simulink model "mrefrobotarm_modified_previous_y_previous_u_previous_ref_prepro"  (R2018b)
settings: Solver=FixedStepAuto  StartTime=0.0  StopTime=10  RelTol=1e-3  AbsTol=1e-6
undefined symbols (not defined in the file or in its folder): cc, options
libraries: neural x594, simulink x1
(part 6 of 22)

== system mrefrobotarm_modified_previous_y_previous_u_previous_ref_prepro/m=0.01 sd =0.01/Layer 3/Delays 1 ==
  "p{3}" : Inport  PortDimensions=30
      mask Display: e = 0.06;c1 = [120 230 180]/255;c2 = ([120 230 180]+0)/(256+128);c3 = ([120 230 180]+128)/(256+128);patch([0 1 1 0],[0 0 1 1],c1);patch([0 1 1 1-e 1-e 0+e],[0 0 1 1-e 0+e 0+e],c2);patch([0 0 1 1-e 0+e 0+e],[0 1 1 1-e 1-e 0+e],c3);plot([0 1 1 0 0],[0 0 1 1 0]);
  mux : Mux  Inputs=1
      mask Display: e = 0.06;c1 = [120 150 230]/255;c2 = ([120 150 230]+0)/383;c3 = ([120 150 230]+128)/383;patch([0 1 1 0],[0 0 1 1],c1);patch([0 1 1 1-e 1-e 0+e],[0 0 1 1-e 0+e 0+e],c2);patch([0 0 1 1-e 0+e 0+e],[0 1 1 1-e 1-e 0+e],c3);plot([0 1 1 0 0],[0 0 1 1 0]);disp('Mux')
  "pd{3,2}" : Outport
      mask Display: e = 0.06;c1 = [120 230 180]/255;c2 = ([120 230 180]+0)/(256+128);c3 = ([120 230 180]+128)/(256+128);patch([0 1 1 0],[0 0 1 1],c1);patch([0 1 1 1-e 1-e 0+e],[0 0 1 1-e 0+e 0+e],c2);patch([0 0 1 1-e 0+e 0+e],[0 1 1 1-e 1-e 0+e],c3);plot([0 1 1 0 0],[0 0 1 1 0]);
  wires:
  "p{3}"/1 -> mux/1
  mux/1 -> "pd{3,2}"/1

== system mrefrobotarm_modified_previous_y_previous_u_previous_ref_prepro/m=0.01 sd =0.01/Layer 3/LW{3,2} ==
  "ad{3,2}" : Inport  PortDimensions=30
      mask Display: e = 0.06;c1 = [120 230 180]/255;c2 = ([120 230 180]+0)/(256+128);c3 = ([120 230 180]+128)/(256+128);patch([0 1 1 0],[0 0 1 1],c1);patch([0 1 1 1-e 1-e 0+e],[0 0 1 1-e 0+e 0+e],c2);patch([0 0 1 1-e 0+e 0+e],[0 1 1 1-e 1-e 0+e],c3);plot([0 1 1 0 0],[0 0 1 1 0]);
  "IW{3,2}(1,:)'" : Constant  Value=[0.0028381381201219024745796559727750718593597412109375;-0.00708260609535531389380214051243456196971237659454345703125;-0.00583488335220346855669593111315407440997660160064697265625;0.01020530930108067869943599959015045897103846073150634765625;0.0035026247420214058798937362126935113337822258472442626953125;0.007372665491954556553355626391521582263521850109100341796875;0.0082512842468972780185509918737807311117649078369140625;-0.006754245741655124334046345069282324402593076229095458984375;0.001683452101721956591096063249324288335628807544708251953125;-0.00690829099421421365112561119303791201673448085784912109375;0.01314880348478297822367721892078407108783721923828125;-0.007470263091506845927469715462621024926193058490753173828125;-0.00542419932097103381363201179965471965260803699493408203125;-0.01146260049752216743368382623202705872245132923126220703125;-0.009116602607925426704493787610772415064275264739990234375;-0.0032803912590090062058323372440327148069627583026885986328125;-0.006661633151908582205213971150215002126060426235198974609375;-0.0289839272926558366716420778175233863294124603271484375;0.007080157965975715332607176577539576101116836071014404296875;1.106395796742202453089021219057030975818634033203125;0.0098157682894019597508172836342055234126746654510498046875;-0.00914110666628639191577665457089096889831125736236572265625;-0.00060787204210546621867272687467220748658291995525360107421875;-0.00883143986489790498717322719812727882526814937591552734375;0.0082676478536601351321255748416660935617983341217041015625;-0.00932936505581516591079083156046181102283298969268798828125;-0.00127195106162408637373584241458956967107951641082763671875;-0.00692592170297301294723535391995028476230800151824951171875;0.009542106880190574791367197349245543591678142547607421875;-0.00879287702148130560775296515885202097706496715545654296875]
      mask Display: e = 0.06;c1 = [120 150 230]/255;c2 = ([120 150 230]+0)/383;c3 = ([120 150 230]+128)/383;patch([0 1 1 0],[0 0 1 1],c1);patch([0 1 1 1-e 1-e 0+e],[0 0 1 1-e 0+e 0+e],c2);patch([0 0 1 1-e 0+e 0+e],[0 1 1 1-e 1-e 0+e],c3);plot([0 1 1 0 0],[0 0 1 1 0]);disp('weights');
  Mux : Mux  Inputs=1
      mask Display: e = 0.06;c1 = [120 150 230]/255;c2 = ([120 150 230]+0)/383;c3 = ([120 150 230]+128)/383;patch([0 1 1 0],[0 0 1 1],c1);patch([0 1 1 1-e 1-e 0+e],[0 0 1 1-e 0+e 0+e],c2);patch([0 0 1 1-e 0+e 0+e],[0 1 1 1-e 1-e 0+e],c3);plot([0 1 1 0 0],[0 0 1 1 0]);disp('Mux');
  dotprod1 : neural/Weight Functions/dotprod
  "lz{3,2}" : Outport
      mask Display: e = 0.06;c1 = [120 230 180]/255;c2 = ([120 230 180]+0)/(256+128);c3 = ([120 230 180]+128)/(256+128);patch([0 1 1 0],[0 0 1 1],c1);patch([0 1 1 1-e 1-e 0+e],[0 0 1 1-e 0+e 0+e],c2);patch([0 0 1 1-e 0+e 0+e],[0 1 1 1-e 1-e 0+e],c3);plot([0 1 1 0 0],[0 0 1 1 0]);
  wires:
  "IW{3,2}(1,:)'"/1 -> dotprod1/1
  "ad{3,2}"/1 -> dotprod1/2
  dotprod1/1 -> Mux/1
  Mux/1 -> "lz{3,2}"/1

== system mrefrobotarm_modified_previous_y_previous_u_previous_ref_prepro/pre_0/Layer 1/Delays 1 ==
  "p{1}" : Inport  PortDimensions=10
      mask Display: e = 0.06;c1 = [120 230 180]/255;c2 = ([120 230 180]+0)/(256+128);c3 = ([120 230 180]+128)/(256+128);patch([0 1 1 0],[0 0 1 1],c1);patch([0 1 1 1-e 1-e 0+e],[0 0 1 1-e 0+e 0+e],c2);patch([0 0 1 1-e 0+e 0+e],[0 1 1 1-e 1-e 0+e],c3);plot([0 1 1 0 0],[0 0 1 1 0]);
  mux : Mux  Inputs=1
      mask Display: e = 0.06;c1 = [120 150 230]/255;c2 = ([120 150 230]+0)/383;c3 = ([120 150 230]+128)/383;patch([0 1 1 0],[0 0 1 1],c1);patch([0 1 1 1-e 1-e 0+e],[0 0 1 1-e 0+e 0+e],c2);patch([0 0 1 1-e 0+e 0+e],[0 1 1 1-e 1-e 0+e],c3);plot([0 1 1 0 0],[0 0 1 1 0]);disp('Mux')
  "pd{1,1}" : Outport
      mask Display: e = 0.06;c1 = [120 230 180]/255;c2 = ([120 230 180]+0)/(256+128);c3 = ([120 230 180]+128)/(256+128);patch([0 1 1 0],[0 0 1 1],c1);patch([0 1 1 1-e 1-e 0+e],[0 0 1 1-e 0+e 0+e],c2);patch([0 0 1 1-e 0+e 0+e],[0 1 1 1-e 1-e 0+e],c3);plot([0 1 1 0 0],[0 0 1 1 0]);
  wires:
  "p{1}"/1 -> mux/1
  mux/1 -> "pd{1,1}"/1

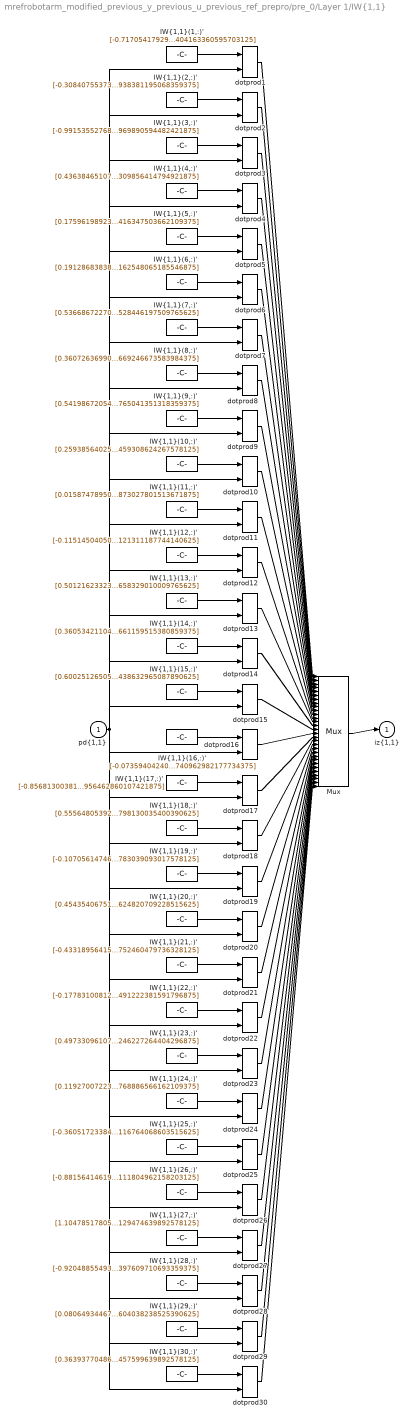
== system mrefrobotarm_modified_previous_y_previous_u_previous_ref_prepro/pre_0/Layer 1/IW{1,1} ==
  "pd{1,1}" : Inport  PortDimensions=10
      mask Display: e = 0.06;c1 = [120 230 180]/255;c2 = ([120 230 180]+0)/(256+128);c3 = ([120 230 180]+128)/(256+128);patch([0 1 1 0],[0 0 1 1],c1);patch([0 1 1 1-e 1-e 0+e],[0 0 1 1-e 0+e 0+e],c2);patch([0 0 1 1-e 0+e 0+e],[0 1 1 1-e 1-e 0+e],c3);plot([0 1 1 0 0],[0 0 1 1 0]);
  "IW{1,1}(1,:)'" : Constant  Value=[-0.7170541792926499180538257860462181270122528076171875;-0.53730470878595426587054362244089134037494659423828125;0.85386649215660692657792196769150905311107635498046875;-0.439278400220474873894005440888577140867710113525390625;0.338061858528379610699943214058293960988521575927734375;0.28368532083581954328366236950387246906757354736328125;-0.961821049186493581828472088091075420379638671875;-0.49782743481612723446261270510149188339710235595703125;-0.0877755253396242662855541993849328719079494476318359375;0.180319748256219380966314247416448779404163360595703125]
      mask Display: e = 0.06;c1 = [120 150 230]/255;c2 = ([120 150 230]+0)/383;c3 = ([120 150 230]+128)/383;patch([0 1 1 0],[0 0 1 1],c1);patch([0 1 1 1-e 1-e 0+e],[0 0 1 1-e 0+e 0+e],c2);patch([0 0 1 1-e 0+e 0+e],[0 1 1 1-e 1-e 0+e],c3);plot([0 1 1 0 0],[0 0 1 1 0]);disp('Weights');
  "IW{1,1}(10,:)'" : Constant  Value=[0.25938564025182764272159374741022475063800811767578125;-0.5066291721836615469243270126753486692905426025390625;0.365194749586469746827077642592485062777996063232421875;0.34016798405581039066447601726395078003406524658203125;0.73685097441923164129917722675600089132785797119140625;0.77610806782460539654522335695219226181507110595703125;-0.89757418772604735668352304855943657457828521728515625;0.30341865744586205000388190455851145088672637939453125;0.4921579361872365776520155122852884232997894287109375;-0.635709476416032703838254747097380459308624267578125]
      mask Display: e = 0.06;c1 = [120 150 230]/255;c2 = ([120 150 230]+0)/383;c3 = ([120 150 230]+128)/383;patch([0 1 1 0],[0 0 1 1],c1);patch([0 1 1 1-e 1-e 0+e],[0 0 1 1-e 0+e 0+e],c2);patch([0 0 1 1-e 0+e 0+e],[0 1 1 1-e 1-e 0+e],c3);plot([0 1 1 0 0],[0 0 1 1 0]);disp('Weights');
  "IW{1,1}(11,:)'" : Constant  Value=[0.015874789502760534853909035746255540288984775543212890625;0.462275145120222108463536869749077595770359039306640625;0.0032692520327777508347411039579810676514171063899993896484375;0.05251953017595435702080663986635045148432254791259765625;0.91141322247884082319302478936151601374149322509765625;-0.79281915938791136522212354975636117160320281982421875;-0.4515989926503818363556774784228764474391937255859375;0.9314165577462818479403949822881259024143218994140625;-0.261347523270411274953772817752906121313571929931640625;-0.10546819823597312903995515398491988889873027801513671875]
      mask Display: e = 0.06;c1 = [120 150 230]/255;c2 = ([120 150 230]+0)/383;c3 = ([120 150 230]+128)/383;patch([0 1 1 0],[0 0 1 1],c1);patch([0 1 1 1-e 1-e 0+e],[0 0 1 1-e 0+e 0+e],c2);patch([0 0 1 1-e 0+e 0+e],[0 1 1 1-e 1-e 0+e],c3);plot([0 1 1 0 0],[0 0 1 1 0]);disp('Weights');
  "IW{1,1}(12,:)'" : Constant  Value=[-0.11514504050898012599279951473363325931131839752197265625;0.813469898806353786113731985096819698810577392578125;0.490011957774175499480406870134174823760986328125;0.164969195990666117612732932684593833982944488525390625;-0.85432220477327092122976637256215326488018035888671875;-0.57011847095452872213883210861240513622760772705078125;0.288064489380212174207684938664897345006465911865234375;0.2419661153783553009244400300303823314607143402099609375;0.311681589957975513360821651076548732817173004150390625;-0.1664504145084248210029187475811340846121311187744140625]
      mask Display: e = 0.06;c1 = [120 150 230]/255;c2 = ([120 150 230]+0)/383;c3 = ([120 150 230]+128)/383;patch([0 1 1 0],[0 0 1 1],c1);patch([0 1 1 1-e 1-e 0+e],[0 0 1 1-e 0+e 0+e],c2);patch([0 0 1 1-e 0+e 0+e],[0 1 1 1-e 1-e 0+e],c3);plot([0 1 1 0 0],[0 0 1 1 0]);disp('Weights');
  "IW{1,1}(13,:)'" : Constant  Value=[0.50121623323530239968448540821555070579051971435546875;-0.7679058675490575414102067952626384794712066650390625;0.2332901346448288670831772151359473355114459991455078125;-0.05845892447780610956531432975680218078196048736572265625;-0.52276177164686721265951518944348208606243133544921875;1.161972018816590068723826334462501108646392822265625;0.10355864424138964963173492606074432842433452606201171875;-0.64286579959598366684758730116300284862518310546875;0.3284995499970400079092769374256022274494171142578125;0.667607800202736800798675176338292658329010009765625]
      mask Display: e = 0.06;c1 = [120 150 230]/255;c2 = ([120 150 230]+0)/383;c3 = ([120 150 230]+128)/383;patch([0 1 1 0],[0 0 1 1],c1);patch([0 1 1 1-e 1-e 0+e],[0 0 1 1-e 0+e 0+e],c2);patch([0 0 1 1-e 0+e 0+e],[0 1 1 1-e 1-e 0+e],c3);plot([0 1 1 0 0],[0 0 1 1 0]);disp('Weights');
  "IW{1,1}(14,:)'" : Constant  Value=[0.36053421104863614399249627240351401269435882568359375;-0.1762721064183007946279957423030282370746135711669921875;0.251082557900824177021803507159347645938396453857421875;0.020135728323763042724170446717835147865116596221923828125;-0.85072127871646829877505524564185179769992828369140625;0.84743056157007234929778860532678663730621337890625;-0.945997916723647858106005514855496585369110107421875;0.94095072199429896642186577082611620426177978515625;-0.249932980099258295059172496621613390743732452392578125;0.2125377599592276067763663149889907799661159515380859375]
      mask Display: e = 0.06;c1 = [120 150 230]/255;c2 = ([120 150 230]+0)/383;c3 = ([120 150 230]+128)/383;patch([0 1 1 0],[0 0 1 1],c1);patch([0 1 1 1-e 1-e 0+e],[0 0 1 1-e 0+e 0+e],c2);patch([0 0 1 1-e 0+e 0+e],[0 1 1 1-e 1-e 0+e],c3);plot([0 1 1 0 0],[0 0 1 1 0]);disp('Weights');
  "IW{1,1}(15,:)'" : Constant  Value=[0.60025126505590609138351965157198719680309295654296875;-0.66688231279006193741309971301234327256679534912109375;-0.91654840056374220491619553286000154912471771240234375;-0.471001673909513030036322334126452915370464324951171875;0.53790409729519372827866163788712583482265472412109375;0.5322213146726231247640725996461696922779083251953125;0.138282833645754166251862216086010448634624481201171875;-0.77416314549115250454036640803678892552852630615234375;-0.5552894515247055462481284848763607442378997802734375;0.1648030102917383832306086333119310438632965087890625]
      mask Display: e = 0.06;c1 = [120 150 230]/255;c2 = ([120 150 230]+0)/383;c3 = ([120 150 230]+128)/383;patch([0 1 1 0],[0 0 1 1],c1);patch([0 1 1 1-e 1-e 0+e],[0 0 1 1-e 0+e 0+e],c2);patch([0 0 1 1-e 0+e 0+e],[0 1 1 1-e 1-e 0+e],c3);plot([0 1 1 0 0],[0 0 1 1 0]);disp('Weights');
  "IW{1,1}(16,:)'" : Constant  Value=[-0.0735940424037289375736037300157477147877216339111328125;0.12992241719517527709371051969355903565883636474609375;0.3713405142616206244809973213705234229564666748046875;0.1763399041436344572009176090432447381317615509033203125;-0.05111110475284337539836343466959078796207904815673828125;0.460151189735468924002503854353562928736209869384765625;0.7322632127881096852917153228190727531909942626953125;-1.007932226242228779256038251332938671112060546875;0.77228494687098148130388608478824608027935028076171875;-0.37142538987047879484038048758520744740962982177734375]
      mask Display: e = 0.06;c1 = [120 150 230]/255;c2 = ([120 150 230]+0)/383;c3 = ([120 150 230]+128)/383;patch([0 1 1 0],[0 0 1 1],c1);patch([0 1 1 1-e 1-e 0+e],[0 0 1 1-e 0+e 0+e],c2);patch([0 0 1 1-e 0+e 0+e],[0 1 1 1-e 1-e 0+e],c3);plot([0 1 1 0 0],[0 0 1 1 0]);disp('Weights');
  "IW{1,1}(17,:)'" : Constant  Value=[-0.85681300381991631898159766933531500399112701416015625;-0.53097179335189592652710643960745073854923248291015625;1.01247292983426628865117891109548509120941162109375;0.378991230739149143058597246636054478585720062255859375;0.294378095574322984351312015860457904636859893798828125;-0.602953992325712562205808353610336780548095703125;-0.56336544113835262947986848303116858005523681640625;0.90595353858253113710219395215972326695919036865234375;0.57769092650718534276421678441693075001239776611328125;0.89314033041056084538666937078232876956462860107421875]
      mask Display: e = 0.06;c1 = [120 150 230]/255;c2 = ([120 150 230]+0)/383;c3 = ([120 150 230]+128)/383;patch([0 1 1 0],[0 0 1 1],c1);patch([0 1 1 1-e 1-e 0+e],[0 0 1 1-e 0+e 0+e],c2);patch([0 0 1 1-e 0+e 0+e],[0 1 1 1-e 1-e 0+e],c3);plot([0 1 1 0 0],[0 0 1 1 0]);disp('Weights');
  "IW{1,1}(18,:)'" : Constant  Value=[0.555648053924087559352074094931595027446746826171875;0.504375695640225440996573524898849427700042724609375;-0.333632718241962333838301901778322644531726837158203125;0.5008843209308257993228608029312454164028167724609375;-0.237702821178001288959791281740763224661350250244140625;-0.7162760582970670864000339861377142369747161865234375;0.51637313021700015358561586253927089273929595947265625;0.173311238874638118279136733690393157303333282470703125;-0.7997650713717643355948894168250262737274169921875;-0.8738812033958078817619252731674350798130035400390625]
      mask Display: e = 0.06;c1 = [120 150 230]/255;c2 = ([120 150 230]+0)/383;c3 = ([120 150 230]+128)/383;patch([0 1 1 0],[0 0 1 1],c1);patch([0 1 1 1-e 1-e 0+e],[0 0 1 1-e 0+e 0+e],c2);patch([0 0 1 1-e 0+e 0+e],[0 1 1 1-e 1-e 0+e],c3);plot([0 1 1 0 0],[0 0 1 1 0]);disp('Weights');
  "IW{1,1}(19,:)'" : Constant  Value=[-0.10705614746581405827274835473872371949255466461181640625;0.1487441877660455047394094663104624487459659576416015625;-0.26390898079033842105189933135989122092723846435546875;-0.6493337689871576667854924380662851035594940185546875;-0.46145541066660289430956254363991320133209228515625;-0.142170787004473997416909014646080322563648223876953125;1.012033043287881017846530085080303251743316650390625;-0.319071927015635414814909154301858507096767425537109375;-0.516709582947004530950607659178785979747772216796875;0.50320529256654034089280003172461874783039093017578125]
      mask Display: e = 0.06;c1 = [120 150 230]/255;c2 = ([120 150 230]+0)/383;c3 = ([120 150 230]+128)/383;patch([0 1 1 0],[0 0 1 1],c1);patch([0 1 1 1-e 1-e 0+e],[0 0 1 1-e 0+e 0+e],c2);patch([0 0 1 1-e 0+e 0+e],[0 1 1 1-e 1-e 0+e],c3);plot([0 1 1 0 0],[0 0 1 1 0]);disp('Weights');
  "IW{1,1}(2,:)'" : Constant  Value=[-0.30840755373511308246037287972285412251949310302734375;-0.099084112890050535238373186075477860867977142333984375;0.81717661091166771125671175468596629798412322998046875;-0.6092062881178741395871156782959587872028350830078125;-0.50860553050792145501901586612802930176258087158203125;-0.6625835472015584315386149683035910129547119140625;0.75851058462894760392458692876971326768398284912109375;-0.037532246529271333368438234856512281112372875213623046875;0.79511476519777823934731486588134430348873138427734375;0.37191656633381453556097540058544836938381195068359375]
      mask Display: e = 0.06;c1 = [120 150 230]/255;c2 = ([120 150 230]+0)/383;c3 = ([120 150 230]+128)/383;patch([0 1 1 0],[0 0 1 1],c1);patch([0 1 1 1-e 1-e 0+e],[0 0 1 1-e 0+e 0+e],c2);patch([0 0 1 1-e 0+e 0+e],[0 1 1 1-e 1-e 0+e],c3);plot([0 1 1 0 0],[0 0 1 1 0]);disp('Weights');
  "IW{1,1}(20,:)'" : Constant  Value=[0.454354067516998527676008734488277696073055267333984375;0.57137295812917321402579773348406888544559478759765625;-0.1850233688088059047505140597422723658382892608642578125;0.386724997843112927586872729079914279282093048095703125;0.039258849478771173924229742624447681009769439697265625;0.67472078143233493729979954878217540681362152099609375;0.92573329751093591521993175774696283042430877685546875;-0.70208984056181711341793061365024186670780181884765625;-0.7554651342448270856522185567882843315601348876953125;-0.653164724819280451129088760353624820709228515625]
      mask Display: e = 0.06;c1 = [120 150 230]/255;c2 = ([120 150 230]+0)/383;c3 = ([120 150 230]+128)/383;patch([0 1 1 0],[0 0 1 1],c1);patch([0 1 1 1-e 1-e 0+e],[0 0 1 1-e 0+e 0+e],c2);patch([0 0 1 1-e 0+e 0+e],[0 1 1 1-e 1-e 0+e],c3);plot([0 1 1 0 0],[0 0 1 1 0]);disp('Weights');
  "IW{1,1}(21,:)'" : Constant  Value=[-0.4331895641543983543897411436773836612701416015625;0.8989764475014252465001618475071154534816741943359375;-0.54666182104691929399820082835503853857517242431640625;-0.56008518072537050169756867035175673663616180419921875;-0.177121978724637030300215201350511051714420318603515625;-0.9354064903881589287948372657410800457000732421875;0.5262284428804051561456844865460880100727081298828125;0.638291312447713199418330987100489437580108642578125;-0.372536639664820812267720384625135920941829681396484375;-0.60323093663160876065632010067929513752460479736328125]
      mask Display: e = 0.06;c1 = [120 150 230]/255;c2 = ([120 150 230]+0)/383;c3 = ([120 150 230]+128)/383;patch([0 1 1 0],[0 0 1 1],c1);patch([0 1 1 1-e 1-e 0+e],[0 0 1 1-e 0+e 0+e],c2);patch([0 0 1 1-e 0+e 0+e],[0 1 1 1-e 1-e 0+e],c3);plot([0 1 1 0 0],[0 0 1 1 0]);disp('Weights');
  "IW{1,1}(22,:)'" : Constant  Value=[-0.1778310081286245125653522336506284773349761962890625;-0.58116958910897731360734042027615942060947418212890625;0.76548783415328924828457957119098864495754241943359375;0.311107618873479319088204420040710829198360443115234375;-0.03968922139101148383044659340157522819936275482177734375;-0.843995838711065093917795820743776857852935791015625;0.206526298912914629823944778763689100742340087890625;-0.359170465722282561404909984048572368919849395751953125;0.5525388023226003308963072413462214171886444091796875;1.0572457569624578166411765778320841491222381591796875]
      mask Display: e = 0.06;c1 = [120 150 230]/255;c2 = ([120 150 230]+0)/383;c3 = ([120 150 230]+128)/383;patch([0 1 1 0],[0 0 1 1],c1);patch([0 1 1 1-e 1-e 0+e],[0 0 1 1-e 0+e 0+e],c2);patch([0 0 1 1-e 0+e 0+e],[0 1 1 1-e 1-e 0+e],c3);plot([0 1 1 0 0],[0 0 1 1 0]);disp('Weights');
  "IW{1,1}(23,:)'" : Constant  Value=[0.49733096107312502187625113947433419525623321533203125;0.89927052734582202386803828630945645272731781005859375;-0.0394225177103877388873343079467304050922393798828125;-0.57836371627708604847839524154551327228546142578125;0.1021461496097287591222624314468703232705593109130859375;0.038811398906852888346374896855195402167737483978271484375;0.2188587004529818080822423098652507178485393524169921875;0.28864377705730703826958460922469384968280792236328125;-0.11510758072953168607011065205369959585368633270263671875;-1.082554482942160500869022143888287246227264404296875]
      mask Display: e = 0.06;c1 = [120 150 230]/255;c2 = ([120 150 230]+0)/383;c3 = ([120 150 230]+128)/383;patch([0 1 1 0],[0 0 1 1],c1);patch([0 1 1 1-e 1-e 0+e],[0 0 1 1-e 0+e 0+e],c2);patch([0 0 1 1-e 0+e 0+e],[0 1 1 1-e 1-e 0+e],c3);plot([0 1 1 0 0],[0 0 1 1 0]);disp('Weights');
  "IW{1,1}(24,:)'" : Constant  Value=[0.11927007223421805248708693625303567387163639068603515625;-0.78217240703766410803154940367676317691802978515625;0.79957722702048228402560425820411182940006256103515625;-0.68075308000872591929208965666475705802440643310546875;0.67785256439370822345580336332204751670360565185546875;-0.46377662029388100339843958863639272749423980712890625;-0.7071229604349558162112998616066761314868927001953125;0.32062142479983446463620566646568477153778076171875;1.0306127438644454574756537112989462912082672119140625;0.474999448772362276027791949672973714768886566162109375]
      mask Display: e = 0.06;c1 = [120 150 230]/255;c2 = ([120 150 230]+0)/383;c3 = ([120 150 230]+128)/383;patch([0 1 1 0],[0 0 1 1],c1);patch([0 1 1 1-e 1-e 0+e],[0 0 1 1-e 0+e 0+e],c2);patch([0 0 1 1-e 0+e 0+e],[0 1 1 1-e 1-e 0+e],c3);plot([0 1 1 0 0],[0 0 1 1 0]);disp('Weights');
  "IW{1,1}(25,:)'" : Constant  Value=[-0.360517233844824591670885638450272381305694580078125;0.626951775382905029943003683001734316349029541015625;-0.8230933590212885508918816412915475666522979736328125;0.328523124878589367625636441516689956188201904296875;0.413636637935129114485022228109301067888736724853515625;-1.035828337086357908702893837471492588520050048828125;0.256185564519046560238990650759660638868808746337890625;0.5580488933457392608517011467483825981616973876953125;0.09104839368044533032264808980471570976078510284423828125;0.67183685486697142241752089830697514116764068603515625]
      mask Display: e = 0.06;c1 = [120 150 230]/255;c2 = ([120 150 230]+0)/383;c3 = ([120 150 230]+128)/383;patch([0 1 1 0],[0 0 1 1],c1);patch([0 1 1 1-e 1-e 0+e],[0 0 1 1-e 0+e 0+e],c2);patch([0 0 1 1-e 0+e 0+e],[0 1 1 1-e 1-e 0+e],c3);plot([0 1 1 0 0],[0 0 1 1 0]);disp('Weights');
  "IW{1,1}(26,:)'" : Constant  Value=[-0.8815641461967269609800723628723062574863433837890625;0.6197700815159847831381512150983326137065887451171875;0.292051004807718450617670669089420698583126068115234375;0.26881320319315460398712502865237183868885040283203125;0.249493533032821790396127425992744974792003631591796875;1.05959018245037395189456219668500125408172607421875;-0.293385437330179354997738983001909218728542327880859375;-0.399771731559667553579373588945600204169750213623046875;-0.34656020453818781046351205077371560037136077880859375;-0.6314877403176819559149635097128339111804962158203125]
      mask Display: e = 0.06;c1 = [120 150 230]/255;c2 = ([120 150 230]+0)/383;c3 = ([120 150 230]+128)/383;patch([0 1 1 0],[0 0 1 1],c1);patch([0 1 1 1-e 1-e 0+e],[0 0 1 1-e 0+e 0+e],c2);patch([0 0 1 1-e 0+e 0+e],[0 1 1 1-e 1-e 0+e],c3);plot([0 1 1 0 0],[0 0 1 1 0]);disp('Weights');
  "IW{1,1}(27,:)'" : Constant  Value=[1.104785178057527961215100731351412832736968994140625;0.92382265168978860980786294021527282893657684326171875;-0.2163549018084075237222663190550520084798336029052734375;-0.9299599360027439587383923935703933238983154296875;1.0641081287763214380248655288596637547016143798828125;-0.431724090480411437642516148116555996239185333251953125;-0.6106446219490513360739214476780034601688385009765625;0.12364313447965613601553513944963924586772918701171875;-0.1852884010195837427570353383998735807836055755615234375;-0.27181446044382007176665183578734286129474639892578125]
      mask Display: e = 0.06;c1 = [120 150 230]/255;c2 = ([120 150 230]+0)/383;c3 = ([120 150 230]+128)/383;patch([0 1 1 0],[0 0 1 1],c1);patch([0 1 1 1-e 1-e 0+e],[0 0 1 1-e 0+e 0+e],c2);patch([0 0 1 1-e 0+e 0+e],[0 1 1 1-e 1-e 0+e],c3);plot([0 1 1 0 0],[0 0 1 1 0]);disp('Weights');
  "IW{1,1}(28,:)'" : Constant  Value=[-0.9204885549329322458333990653045475482940673828125;0.71505473712299216781929089847835712134838104248046875;0.1774163810718654421538786891687777824699878692626953125;-0.26649356933898171728714032724383287131786346435546875;0.00214973842263012186737380915246831136755645275115966796875;0.74548203298877979694481155092944391071796417236328125;-0.1985219038956410886331838128171511925756931304931640625;-0.59169123834156944763407182108494453132152557373046875;0.63985644297602572994065894818049855530261993408203125;-0.76998465204601840294884596005431376397609710693359375]
      mask Display: e = 0.06;c1 = [120 150 230]/255;c2 = ([120 150 230]+0)/383;c3 = ([120 150 230]+128)/383;patch([0 1 1 0],[0 0 1 1],c1);patch([0 1 1 1-e 1-e 0+e],[0 0 1 1-e 0+e 0+e],c2);patch([0 0 1 1-e 0+e 0+e],[0 1 1 1-e 1-e 0+e],c3);plot([0 1 1 0 0],[0 0 1 1 0]);disp('Weights');
  "IW{1,1}(29,:)'" : Constant  Value=[0.08064934467823166308608762165022199042141437530517578125;-0.51833738280565244682662751074531115591526031494140625;-0.652571486768099617847838089801371097564697265625;-0.6650816931740599624589549421216361224651336669921875;0.428389676123669571605745431952527724206447601318359375;0.5646866986895844320315518416464328765869140625;-0.334055174362817230981903549036360345780849456787109375;-0.35511580527712072186119485195376910269260406494140625;0.376377376211224301538749159590224735438823699951171875;0.97045606723925426084775835988693870604038238525390625]
      mask Display: e = 0.06;c1 = [120 150 230]/255;c2 = ([120 150 230]+0)/383;c3 = ([120 150 230]+128)/383;patch([0 1 1 0],[0 0 1 1],c1);patch([0 1 1 1-e 1-e 0+e],[0 0 1 1-e 0+e 0+e],c2);patch([0 0 1 1-e 0+e 0+e],[0 1 1 1-e 1-e 0+e],c3);plot([0 1 1 0 0],[0 0 1 1 0]);disp('Weights');
  "IW{1,1}(3,:)'" : Constant  Value=[-0.99153552768192054767126819569966755807399749755859375;0.64787754216170279075726057271822355687618255615234375;0.68028029231688569300473545808927156031131744384765625;-0.69196568392561663696227469699806533753871917724609375;0.1267368240162062564824196897461661137640476226806640625;-0.43286605744731165845706755135324783623218536376953125;-0.467372693569951980219201459476607851684093475341796875;0.427710043483989277302015352688613347709178924560546875;0.334351945503890080058084777192561887204647064208984375;0.056962416338333481113931355821478064171969890594482421875]
      mask Display: e = 0.06;c1 = [120 150 230]/255;c2 = ([120 150 230]+0)/383;c3 = ([120 150 230]+128)/383;patch([0 1 1 0],[0 0 1 1],c1);patch([0 1 1 1-e 1-e 0+e],[0 0 1 1-e 0+e 0+e],c2);patch([0 0 1 1-e 0+e 0+e],[0 1 1 1-e 1-e 0+e],c3);plot([0 1 1 0 0],[0 0 1 1 0]);disp('Weights');
  "IW{1,1}(30,:)'" : Constant  Value=[0.363937704867758615723261073071626015007495880126953125;0.30746852825596071578928558665211312472820281982421875;0.08207578531167457336348292074035271070897579193115234375;0.74981417951573192670622347577591426670551300048828125;-0.46676131123100528252933827388915233314037322998046875;-0.74448595717461873988440856919623911380767822265625;-0.1715609051203128843088308030928601510822772979736328125;-0.6088199470498143472951824151095934212207794189453125;-0.7969457614862556216195343949948437511920928955078125;-0.02125102504300242778345619854007964022457599639892578125]
      mask Display: e = 0.06;c1 = [120 150 230]/255;c2 = ([120 150 230]+0)/383;c3 = ([120 150 230]+128)/383;patch([0 1 1 0],[0 0 1 1],c1);patch([0 1 1 1-e 1-e 0+e],[0 0 1 1-e 0+e 0+e],c2);patch([0 0 1 1-e 0+e 0+e],[0 1 1 1-e 1-e 0+e],c3);plot([0 1 1 0 0],[0 0 1 1 0]);disp('Weights');
  "IW{1,1}(4,:)'" : Constant  Value=[0.43638465107237267570639005498378537595272064208984375;0.4617365655073857322321373430895619094371795654296875;-0.326678405985217690243871402344666421413421630859375;0.292387559672311170277936298589338548481464385986328125;0.68565165583534815052502153776003979146480560302734375;-0.8202765637128610620720792212523519992828369140625;-0.01647018295307640933788917436686460860073566436767578125;-0.766025218483262992918980671674944460391998291015625;-0.52751398826329509716970278532244265079498291015625;0.8377487697174792469212434298242442309856414794921875]
      mask Display: e = 0.06;c1 = [120 150 230]/255;c2 = ([120 150 230]+0)/383;c3 = ([120 150 230]+128)/383;patch([0 1 1 0],[0 0 1 1],c1);patch([0 1 1 1-e 1-e 0+e],[0 0 1 1-e 0+e 0+e],c2);patch([0 0 1 1-e 0+e 0+e],[0 1 1 1-e 1-e 0+e],c3);plot([0 1 1 0 0],[0 0 1 1 0]);disp('Weights');
  "IW{1,1}(5,:)'" : Constant  Value=[0.1759619892392587925389335623549413867294788360595703125;0.7696542440388987049715296961949206888675689697265625;-0.851376287127035613622183518600650131702423095703125;0.5058989985838786562766244969679974019527435302734375;-0.68537890003123680404684137101867236196994781494140625;0.73742092979006124142671296795015223324298858642578125;-0.54409406720694641901303612030460499227046966552734375;0.53784386928414285033994701734627597033977508544921875;0.23237060543502685572292421056772582232952117919921875;0.6989266223128784982776551260030828416347503662109375]
      mask Display: e = 0.06;c1 = [120 150 230]/255;c2 = ([120 150 230]+0)/383;c3 = ([120 150 230]+128)/383;patch([0 1 1 0],[0 0 1 1],c1);patch([0 1 1 1-e 1-e 0+e],[0 0 1 1-e 0+e 0+e],c2);patch([0 0 1 1-e 0+e 0+e],[0 1 1 1-e 1-e 0+e],c3);plot([0 1 1 0 0],[0 0 1 1 0]);disp('Weights');
  "IW{1,1}(6,:)'" : Constant  Value=[0.1912868383813841888230200538600911386311054229736328125;-0.9883987240949829722325148395611904561519622802734375;0.28280396803305885011781128923757933080196380615234375;0.333695039449705410650182102472172118723392486572265625;-1.2171952045291052346698279507108964025974273681640625;0.9168264557199308217860789227415807545185089111328125;-0.005957496462494403510756768582723452709615230560302734375;0.64804869858626512613142267582588829100131988525390625;-0.1744585928343133918172469520868617109954357147216796875;-0.3567048492913027502027034643106162548065185546875]
      mask Display: e = 0.06;c1 = [120 150 230]/255;c2 = ([120 150 230]+0)/383;c3 = ([120 150 230]+128)/383;patch([0 1 1 0],[0 0 1 1],c1);patch([0 1 1 1-e 1-e 0+e],[0 0 1 1-e 0+e 0+e],c2);patch([0 0 1 1-e 0+e 0+e],[0 1 1 1-e 1-e 0+e],c3);plot([0 1 1 0 0],[0 0 1 1 0]);disp('Weights');
  "IW{1,1}(7,:)'" : Constant  Value=[0.53668672270431472259843985739280469715595245361328125;-0.86597864285057213340479620455880649387836456298828125;0.367948251905165946151754496895591728389263153076171875;-0.101552911108880816737354280121508054435253143310546875;-0.69480073485182802794923873079824261367321014404296875;0.2886913663394512497006871853955090045928955078125;0.50312288016138906332486158134997822344303131103515625;-0.0504379313138109408587439475013525225222110748291015625;-0.1604759973009884654882029053624137304723262786865234375;0.3626860900910051643819542732671834528446197509765625]
      mask Display: e = 0.06;c1 = [120 150 230]/255;c2 = ([120 150 230]+0)/383;c3 = ([120 150 230]+128)/383;patch([0 1 1 0],[0 0 1 1],c1);patch([0 1 1 1-e 1-e 0+e],[0 0 1 1-e 0+e 0+e],c2);patch([0 0 1 1-e 0+e 0+e],[0 1 1 1-e 1-e 0+e],c3);plot([0 1 1 0 0],[0 0 1 1 0]);disp('Weights');
  "IW{1,1}(8,:)'" : Constant  Value=[0.360726369903551946638486924712196923792362213134765625;-0.772878002787770856940596786444075405597686767578125;0.5845611294740591379337502075941301882266998291015625;-0.432191320709908899377893476412282325327396392822265625;-0.143959327034458295369034885879955254495143890380859375;0.1901128979977855515404172592752729542553424835205078125;-0.73119761460990184698260918594314716756343841552734375;-0.334110543584279995332764201521058566868305206298828125;-0.64012032989790135228957979052211157977581024169921875;0.59361462468974168782409606137662194669246673583984375]
      mask Display: e = 0.06;c1 = [120 150 230]/255;c2 = ([120 150 230]+0)/383;c3 = ([120 150 230]+128)/383;patch([0 1 1 0],[0 0 1 1],c1);patch([0 1 1 1-e 1-e 0+e],[0 0 1 1-e 0+e 0+e],c2);patch([0 0 1 1-e 0+e 0+e],[0 1 1 1-e 1-e 0+e],c3);plot([0 1 1 0 0],[0 0 1 1 0]);disp('Weights');
  "IW{1,1}(9,:)'" : Constant  Value=[0.5419867205458837045028985812678001821041107177734375;-0.37716268711213540854032544302754104137420654296875;0.60587106248181232803773355044540949165821075439453125;-0.94828978630924876114249855163507163524627685546875;0.7741540673161868557627940390375442802906036376953125;-0.33112035983088927704187653944245539605617523193359375;-0.74215804637538818067099555264576338231563568115234375;-0.0184491438498242121823977868189103901386260986328125;0.07912831907276270115847438546552439220249652862548828125;0.540592661988623657265407018712721765041351318359375]
      mask Display: e = 0.06;c1 = [120 150 230]/255;c2 = ([120 150 230]+0)/383;c3 = ([120 150 230]+128)/383;patch([0 1 1 0],[0 0 1 1],c1);patch([0 1 1 1-e 1-e 0+e],[0 0 1 1-e 0+e 0+e],c2);patch([0 0 1 1-e 0+e 0+e],[0 1 1 1-e 1-e 0+e],c3);plot([0 1 1 0 0],[0 0 1 1 0]);disp('Weights');
  Mux : Mux  Inputs=30
      mask Display: e = 0.06;c1 = [120 150 230]/255;c2 = ([120 150 230]+0)/383;c3 = ([120 150 230]+128)/383;patch([0 1 1 0],[0 0 1 1],c1);patch([0 1 1 1-e 1-e 0+e],[0 0 1 1-e 0+e 0+e],c2);patch([0 0 1 1-e 0+e 0+e],[0 1 1 1-e 1-e 0+e],c3);plot([0 1 1 0 0],[0 0 1 1 0]);disp('Mux');
  dotprod{1..30} (30 alike) : neural/Weight Functions/dotprod
  "iz{1,1}" : Outport
      mask Display: e = 0.06;c1 = [120 230 180]/255;c2 = ([120 230 180]+0)/(256+128);c3 = ([120 230 180]+128)/(256+128);patch([0 1 1 0],[0 0 1 1],c1);patch([0 1 1 1-e 1-e 0+e],[0 0 1 1-e 0+e 0+e],c2);patch([0 0 1 1-e 0+e 0+e],[0 1 1 1-e 1-e 0+e],c3);plot([0 1 1 0 0],[0 0 1 1 0]);
  wires:
  "IW{1,1}(1,:)'"/1 -> dotprod1/1
  "pd{1,1}"/1 -> dotprod1/2, dotprod2/2, dotprod3/2, dotprod4/2, dotprod5/2, dotprod6/2, dotprod7/2, dotprod8/2, dotprod9/2, dotprod10/2, dotprod11/2, dotprod12/2, dotprod13/2, dotprod14/2, dotprod15/2, dotprod16/2, dotprod17/2, dotprod18/2, dotprod19/2, dotprod20/2, dotprod21/2, dotprod22/2, dotprod23/2, dotprod24/2, dotprod25/2, dotprod26/2, dotprod27/2, dotprod28/2, dotprod29/2, dotprod30/2
  dotprod1/1 -> Mux/1
  "IW{1,1}(2,:)'"/1 -> dotprod2/1
  dotprod2/1 -> Mux/2
  "IW{1,1}(3,:)'"/1 -> dotprod3/1
  dotprod3/1 -> Mux/3
  "IW{1,1}(4,:)'"/1 -> dotprod4/1
  dotprod4/1 -> Mux/4
  "IW{1,1}(5,:)'"/1 -> dotprod5/1
  dotprod5/1 -> Mux/5
  "IW{1,1}(6,:)'"/1 -> dotprod6/1
  dotprod6/1 -> Mux/6
  "IW{1,1}(7,:)'"/1 -> dotprod7/1
  dotprod7/1 -> Mux/7
  "IW{1,1}(8,:)'"/1 -> dotprod8/1
  dotprod8/1 -> Mux/8
  "IW{1,1}(9,:)'"/1 -> dotprod9/1
  dotprod9/1 -> Mux/9
  "IW{1,1}(10,:)'"/1 -> dotprod10/1
  dotprod10/1 -> Mux/10
  "IW{1,1}(11,:)'"/1 -> dotprod11/1
  dotprod11/1 -> Mux/11
  "IW{1,1}(12,:)'"/1 -> dotprod12/1
  dotprod12/1 -> Mux/12
  "IW{1,1}(13,:)'"/1 -> dotprod13/1
  dotprod13/1 -> Mux/13
  "IW{1,1}(14,:)'"/1 -> dotprod14/1
  dotprod14/1 -> Mux/14
  "IW{1,1}(15,:)'"/1 -> dotprod15/1
  dotprod15/1 -> Mux/15
  "IW{1,1}(16,:)'"/1 -> dotprod16/1
  dotprod16/1 -> Mux/16
  "IW{1,1}(17,:)'"/1 -> dotprod17/1
  dotprod17/1 -> Mux/17
  "IW{1,1}(18,:)'"/1 -> dotprod18/1
  dotprod18/1 -> Mux/18
  "IW{1,1}(19,:)'"/1 -> dotprod19/1
  dotprod19/1 -> Mux/19
  "IW{1,1}(20,:)'"/1 -> dotprod20/1
  dotprod20/1 -> Mux/20
  "IW{1,1}(21,:)'"/1 -> dotprod21/1
  dotprod21/1 -> Mux/21
  "IW{1,1}(22,:)'"/1 -> dotprod22/1
  dotprod22/1 -> Mux/22
  "IW{1,1}(23,:)'"/1 -> dotprod23/1
  dotprod23/1 -> Mux/23
  "IW{1,1}(24,:)'"/1 -> dotprod24/1
  dotprod24/1 -> Mux/24
  "IW{1,1}(25,:)'"/1 -> dotprod25/1
  dotprod25/1 -> Mux/25
  "IW{1,1}(26,:)'"/1 -> dotprod26/1
  dotprod26/1 -> Mux/26
  "IW{1,1}(27,:)'"/1 -> dotprod27/1
  dotprod27/1 -> Mux/27
  "IW{1,1}(28,:)'"/1 -> dotprod28/1
  dotprod28/1 -> Mux/28
  "IW{1,1}(29,:)'"/1 -> dotprod29/1
  dotprod29/1 -> Mux/29
  "IW{1,1}(30,:)'"/1 -> dotprod30/1
  dotprod30/1 -> Mux/30
  Mux/1 -> "iz{1,1}"/1

== system mrefrobotarm_modified_previous_y_previous_u_previous_ref_prepro/pre_0/Layer 2/Delays 1 ==
  "p{2}" : Inport  PortDimensions=30
      mask Display: e = 0.06;c1 = [120 230 180]/255;c2 = ([120 230 180]+0)/(256+128);c3 = ([120 230 180]+128)/(256+128);patch([0 1 1 0],[0 0 1 1],c1);patch([0 1 1 1-e 1-e 0+e],[0 0 1 1-e 0+e 0+e],c2);patch([0 0 1 1-e 0+e 0+e],[0 1 1 1-e 1-e 0+e],c3);plot([0 1 1 0 0],[0 0 1 1 0]);
  mux : Mux  Inputs=1
      mask Display: e = 0.06;c1 = [120 150 230]/255;c2 = ([120 150 230]+0)/383;c3 = ([120 150 230]+128)/383;patch([0 1 1 0],[0 0 1 1],c1);patch([0 1 1 1-e 1-e 0+e],[0 0 1 1-e 0+e 0+e],c2);patch([0 0 1 1-e 0+e 0+e],[0 1 1 1-e 1-e 0+e],c3);plot([0 1 1 0 0],[0 0 1 1 0]);disp('Mux')
  "pd{2,1}" : Outport
      mask Display: e = 0.06;c1 = [120 230 180]/255;c2 = ([120 230 180]+0)/(256+128);c3 = ([120 230 180]+128)/(256+128);patch([0 1 1 0],[0 0 1 1],c1);patch([0 1 1 1-e 1-e 0+e],[0 0 1 1-e 0+e 0+e],c2);patch([0 0 1 1-e 0+e 0+e],[0 1 1 1-e 1-e 0+e],c3);plot([0 1 1 0 0],[0 0 1 1 0]);
  wires:
  "p{2}"/1 -> mux/1
  mux/1 -> "pd{2,1}"/1
